simulink library "Process"  (Simulink 10.3)
settings: Solver=ode45  StartTime=0.0  StopTime=10.0  RelTol=1e-3  EnableMultiTasking=on
values from neighbouring files (symbols this model uses):
  Ts = 1    [stepDV.mat]    (also in stepMV.mat; step_MV.mat)
undefined symbols (not defined in the file or in its folder): Kd, Kp, offset_WP, T1, T1d, T2, T2d, theta, thetad
libraries: $bdroot x1, realtime_pacer_lib x1
settings Model: Creator=DBR  LastModifiedBy=thibaut  MultithreadedSim=on

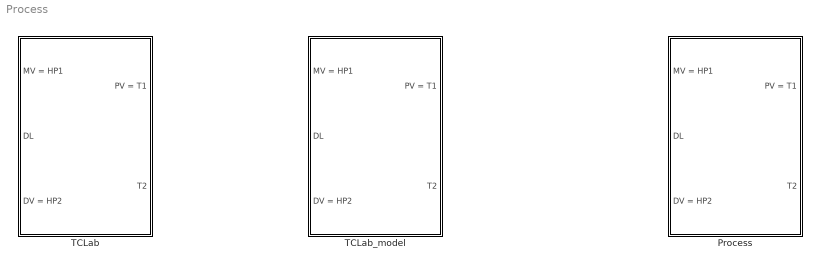
== system Process ==
  Process : Subsystem  BlockChoice=TCLab
      settings: TemplateBlock=self  MemberBlocks=TCLab,TCLab_model
  TCLab : Subsystem
  TCLab_model : Subsystem

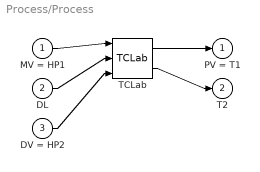
== system Process/Process ==
  MV = HP1 : Inport
  DL : Inport  Port=2
  DV = HP2 : Inport  Port=3
  TCLab : $bdroot/TCLab  SystemSampleTime=-1  VariantActivationTime=update diagram  Latency=0  AutoFrameSizeCalculation=off
  PV = T1 : Outport  VectorParamsAs1DForOutWhenUnconnected=off
  T2 : Outport  Port=2  VectorParamsAs1DForOutWhenUnconnected=off
  wires:
  MV = HP1/1 -> TCLab/1
  DL/1 -> TCLab/2
  DV = HP2/1 -> TCLab/3
  TCLab/1 -> PV = T1/1
  TCLab/2 -> T2/1

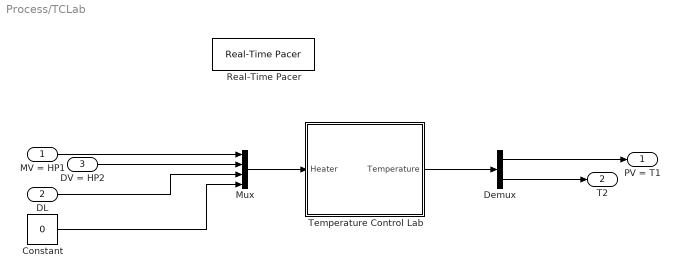
== system Process/TCLab ==
  MV = HP1 : Inport
  DL : Inport  Port=2
  DV = HP2 : Inport  Port=3
  Constant : Constant  Value=0
  Demux : Demux  Outputs=2
  Mux : Mux
  Real-Time Pacer : realtime_pacer_lib/Real-Time Pacer  simTimePerRealTime=1
  Temperature Control Lab : Subsystem
      mask Display: image('tclab.png');
  PV = T1 : Outport  VectorParamsAs1DForOutWhenUnconnected=off
  T2 : Outport  Port=2  VectorParamsAs1DForOutWhenUnconnected=off
  wires:
  MV = HP1/1 -> Mux/1
  DV = HP2/1 -> Mux/2
  Demux/1 -> PV = T1/1
  Demux/2 -> T2/1
  Mux/1 -> Temperature Control Lab/1(Heater)
  Temperature Control Lab/1(Temperature) -> Demux/1
  DL/1 -> Mux/3
  Constant/1 -> Mux/4

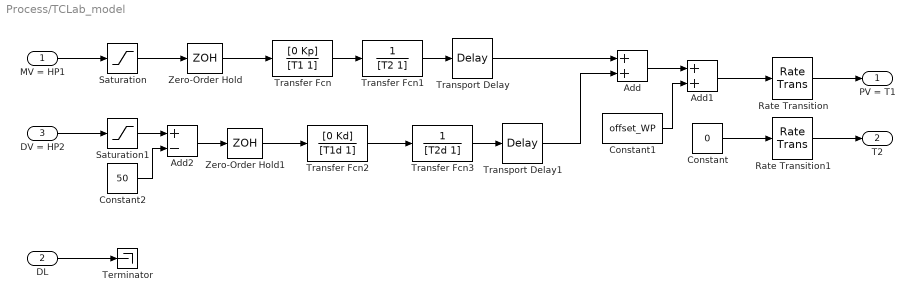
== system Process/TCLab_model ==
  MV = HP1 : Inport
  DL : Inport  Port=2
  DV = HP2 : Inport  Port=3
  Add : Sum
  Add1 : Sum
  Add2 : Sum  Inputs=+-
  Constant : Constant  Value=0
  Constant1 : Constant  Value=offset_WP
  Constant2 : Constant  Value=50
  Rate Transition : RateTransition  OutPortSampleTime=Ts
  Rate Transition1 : RateTransition  OutPortSampleTime=Ts
  Saturation : Saturate  UpperLimit=100  LowerLimit=0
  Saturation1 : Saturate  UpperLimit=100  LowerLimit=0
  Terminator : Terminator
  Transfer Fcn : TransferFcn  Numerator=[0 Kp]  Denominator=[T1 1]
  Transfer Fcn1 : TransferFcn  Numerator=[0 1]  Denominator=[T2 1]
  Transfer Fcn2 : TransferFcn  Numerator=[0 Kd]  Denominator=[T1d 1]
  Transfer Fcn3 : TransferFcn  Numerator=[0 1]  Denominator=[T2d 1]
  Transport Delay : TransportDelay  DelayTime=theta
  Transport Delay1 : TransportDelay  DelayTime=thetad
  Zero-Order Hold : ZeroOrderHold  SampleTime=Ts
  Zero-Order Hold1 : ZeroOrderHold  SampleTime=Ts
  PV = T1 : Outport  VectorParamsAs1DForOutWhenUnconnected=off
  T2 : Outport  Port=2  VectorParamsAs1DForOutWhenUnconnected=off
  wires:
  Saturation/1 -> Zero-Order Hold/1
  Transfer Fcn/1 -> Transfer Fcn1/1
  Zero-Order Hold/1 -> Transfer Fcn/1
  MV = HP1/1 -> Saturation/1
  Transfer Fcn1/1 -> Transport Delay/1
  Transport Delay/1 -> Add/1
  Add/1 -> Add1/1
  Add1/1 -> Rate Transition/1
  Rate Transition/1 -> PV = T1/1
  DV = HP2/1 -> Saturation1/1
  Add2/1 -> Zero-Order Hold1/1
  Saturation1/1 -> Add2/1
  Zero-Order Hold1/1 -> Transfer Fcn2/1
  Transfer Fcn2/1 -> Transfer Fcn3/1
  Transfer Fcn3/1 -> Transport Delay1/1
  Transport Delay1/1 -> Add/2
  Rate Transition1/1 -> T2/1
  Constant/1 -> Rate Transition1/1
  Constant1/1 -> Add1/2
  Constant2/1 -> Add2/2
  DL/1 -> Terminator/1

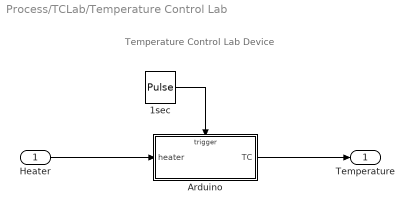
== system Process/TCLab/Temperature Control Lab ==
  note: Temperature Control Lab Device
  Heater : Inport
  1sec : DiscretePulseGenerator  PulseType=Time based  Period=Ts  PulseWidth=50
  Arduino : Subsystem  TreatAsAtomicUnit=on
  Temperature : Outport  VectorParamsAs1DForOutWhenUnconnected=off
  wires:
  1sec/1 -> Arduino/Trigger
  Arduino/1(TC) -> Temperature/1
  Heater/1 -> Arduino/1(heater)

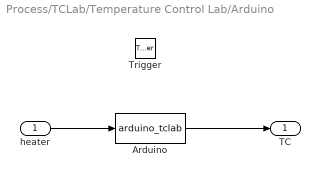
== system Process/TCLab/Temperature Control Lab/Arduino ==
  heater : Inport  LatchByDelayingOutsideSignal=on
  Trigger : TriggerPort  VariantControl=Variant
  Arduino : MATLABFcn  MATLABFcn=arduino_tclab
  TC : Outport  InitialOutput=[23 23]  VectorParamsAs1DForOutWhenUnconnected=off
  wires:
  heater/1 -> Arduino/1
  Arduino/1 -> TC/1
